simulink model "pendulum"  (R2020b)
settings: Solver=ode45  StartTime=0.0  StopTime=10.0  MaxStep=0.01  RelTol=1e-3  EnableMultiTasking=on
values from neighbouring files (symbols this model uses):
  d = 0.2    [init_pendulum.m]
  g = 9.81    [init_pendulum.m]
  l = 1.5    [init_pendulum.m]
  m = 0.5    [init_pendulum.m]
  phi_0 = 178 / 180 * pi    (= 3.10668606855)    [init_pendulum.m]
  phi_dot_0 = 0    [init_pendulum.m]
settings Model: Creator=Goettlicher  LastModifiedBy=60251
settings DataIOCC: LimitDataPoints=on  ReturnWorkspaceOutputs=off
settings OptimizationCC: LifeSpan=inf
settings DebuggingCC: SignalLabelMismatchMsg=error  BusObjectLabelMismatch=error  RootOutportRequireBusObject=error  AllowSymbolicDim=off  SFUnexpectedBacktrackingDiag=warning  SFNoUnconditionalDefaultTransitionDiag=warning  SFExecutionAtInitializationDiag=none  ArithmeticOperatorsInVariantConditions=warning
settings ModelReferenceCC: PropagateSignalLabelsOutOfModel=off
settings SFSimCC: SimUseLocalCustomCode=off  CustomCodeUndefinedFunction=UseInterfaceOnly
settings RTWCC: RTWUseLocalCustomCode=off
settings CodeAppCC: StateflowObjectComments=on
settings GRTTargetCC: TargetLangStandard=C89/C90 (ANSI)
settings ConfigComp: CovMetricSettings=dw  CovSaveCumulativeToWorkspaceVar=on  CovSaveSingleToWorkspaceVar=on  CovExternalEMLEnable=off

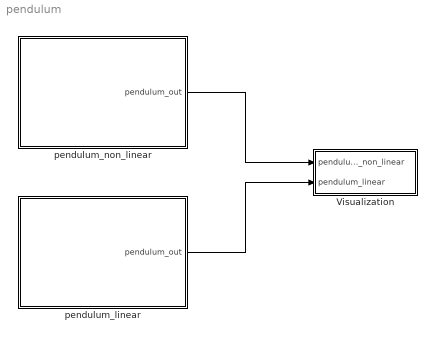
== system pendulum ==
  Visualization : Subsystem
  pendulum_linear : Subsystem
  pendulum_non_linear : Subsystem
  wires:
  pendulum_non_linear/1(pendulum_out) -> Visualization/1(pendulum_non_linear)
  pendulum_linear/1(pendulum_out) -> Visualization/2(pendulum_linear)

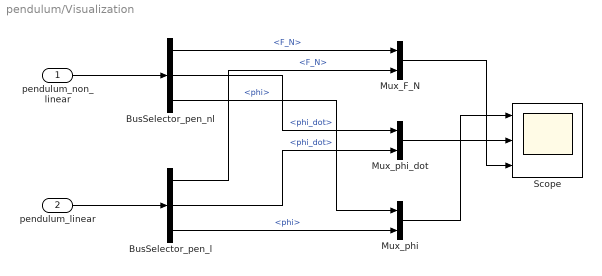
== system pendulum/Visualization ==
  pendulum_non_linear : Inport  OutDataTypeStr=Bus: pendulum_bus
  pendulum_linear : Inport  Port=2  OutDataTypeStr=Bus: pendulum_bus
  BusSelector_pen_l : BusSelector  OutputSignals=F_N,phi_dot,phi
  BusSelector_pen_nl : BusSelector  OutputSignals=F_N,phi_dot,phi
  Mux_F_N : Mux  Inputs=2
  Mux_phi : Mux  Inputs=2
  Mux_phi_dot : Mux  Inputs=2
  Scope : Scope  NumInputPorts=3
  wires:
  pendulum_non_linear/1 -> BusSelector_pen_nl/1
  Mux_phi_dot/1 -> Scope/2
  Mux_F_N/1 -> Scope/3
  Mux_phi/1 -> Scope/1
  pendulum_linear/1 -> BusSelector_pen_l/1
  BusSelector_pen_nl/1 -> Mux_F_N/1  "<F_N>"
  BusSelector_pen_l/1 -> Mux_F_N/2  "<F_N>"
  BusSelector_pen_l/3 -> Mux_phi/2  "<phi>"
  BusSelector_pen_nl/3 -> Mux_phi/1  "<phi>"
  BusSelector_pen_nl/2 -> Mux_phi_dot/1  "<phi_dot>"
  BusSelector_pen_l/2 -> Mux_phi_dot/2  "<phi_dot>"

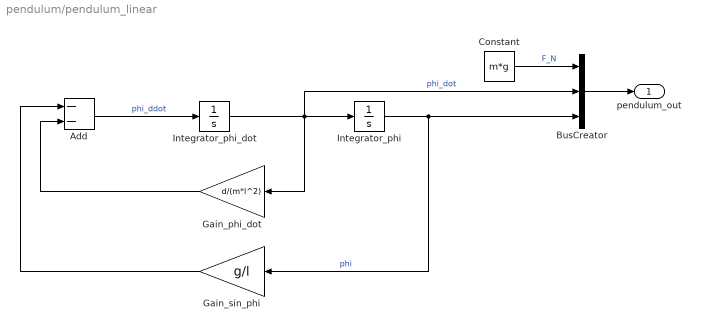
== system pendulum/pendulum_linear ==
  Add : Sum  Inputs=--
  BusCreator : BusCreator  Inputs=3  OutDataTypeStr=Bus: pendulum_bus
  Constant : Constant  Value=m*g
  Gain_phi_dot : Gain  Gain=d/(m*l^2)
  Gain_sin_phi : Gain  Gain=g/l
  Integrator_phi : Integrator  InitialCondition=phi_0
  Integrator_phi_dot : Integrator  InitialCondition=phi_dot_0
  pendulum_out : Outport  OutDataTypeStr=Bus: pendulum_bus
  wires:
  Constant/1 -> BusCreator/1  "F_N"
  Gain_sin_phi/1 -> Add/1
  Integrator_phi/1 -> Gain_sin_phi/1, BusCreator/3  "phi"
  Gain_phi_dot/1 -> Add/2
  Add/1 -> Integrator_phi_dot/1  "phi_ddot"
  Integrator_phi_dot/1 -> BusCreator/2, Gain_phi_dot/1, Integrator_phi/1  "phi_dot"
  BusCreator/1 -> pendulum_out/1

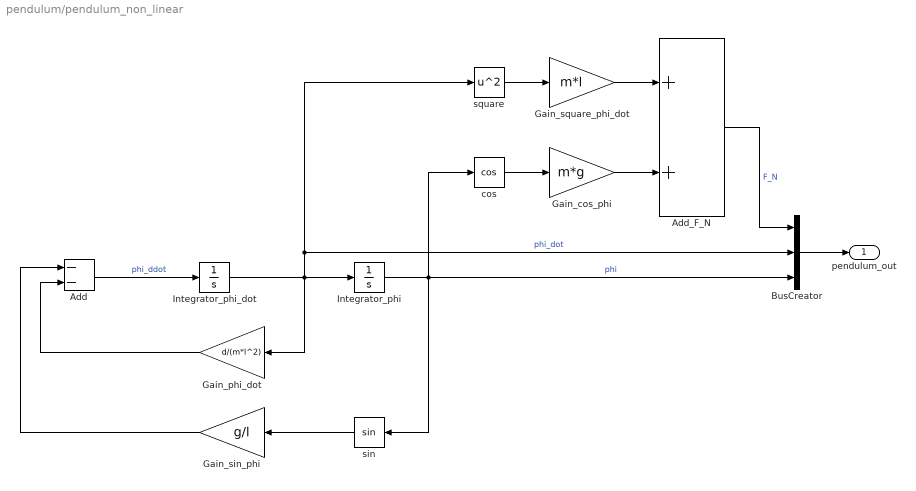
== system pendulum/pendulum_non_linear ==
  Add : Sum  Inputs=--
  Add_F_N : Sum
  BusCreator : BusCreator  Inputs=3  OutDataTypeStr=Bus: pendulum_bus
  Gain_cos_phi : Gain  Gain=m*g
  Gain_phi_dot : Gain  Gain=d/(m*l^2)
  Gain_sin_phi : Gain  Gain=g/l
  Gain_square_phi_dot : Gain  Gain=m*l
  Integrator_phi : Integrator  InitialCondition=phi_0
  Integrator_phi_dot : Integrator  InitialCondition=phi_dot_0
  cos : Trigonometry  Operator=cos
  sin : Trigonometry
  square : Math  Operator=square  SaturateOnIntegerOverflow=on
  pendulum_out : Outport  OutDataTypeStr=Bus: pendulum_bus
  wires:
  BusCreator/1 -> pendulum_out/1
  Integrator_phi_dot/1 -> square/1, BusCreator/2, Gain_phi_dot/1, Integrator_phi/1  "phi_dot"
  Add/1 -> Integrator_phi_dot/1  "phi_ddot"
  Gain_phi_dot/1 -> Add/2
  Integrator_phi/1 -> cos/1, sin/1, BusCreator/3  "phi"
  sin/1 -> Gain_sin_phi/1
  Gain_sin_phi/1 -> Add/1
  Gain_square_phi_dot/1 -> Add_F_N/1
  Gain_cos_phi/1 -> Add_F_N/2
  cos/1 -> Gain_cos_phi/1
  square/1 -> Gain_square_phi_dot/1
  Add_F_N/1 -> BusCreator/1  "F_N"
